simulink model "progetto_smartfarm_luciabrando"  (R2023b)
settings: Solver=VariableStepAuto  StartTime=0.0  StopTime=86400  RelTol=1e-3
libraries: simulink x1
settings Model: Creator=lucia  LastModifiedBy=lucia

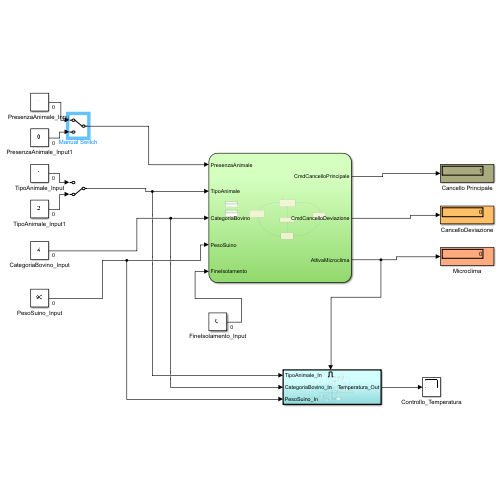
[thumbnail: Simulink's stored preview of the top-level diagram]
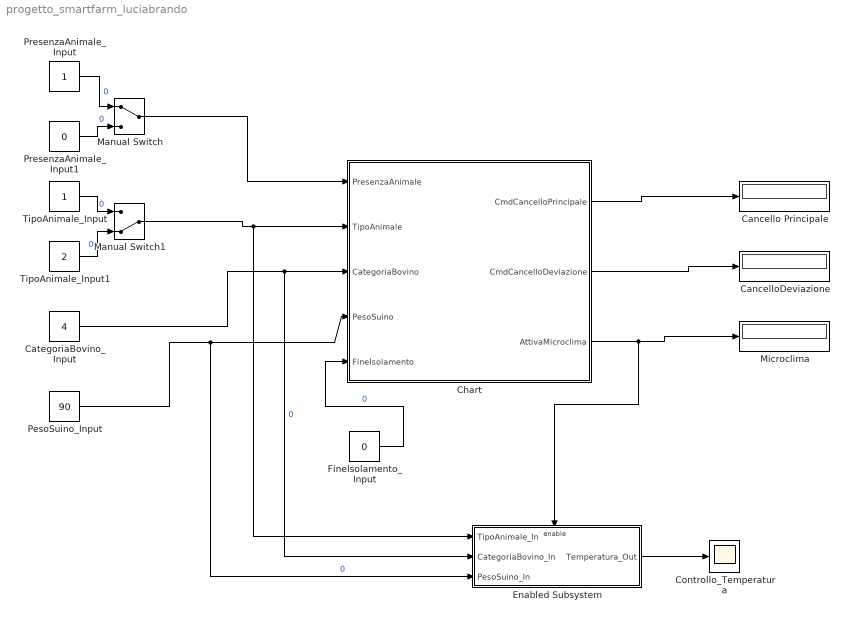
== system progetto_smartfarm_luciabrando ==
  Cancello Principale : Display
  CancelloDeviazione : Display
  CategoriaBovino_Input : Constant  Value=4  OutDataTypeStr=int32
  Chart : Stateflow chart  TreatAsAtomicUnit=on
  Controllo_Temperatura : Scope
  Enabled Subsystem : Subsystem  TreatAsAtomicUnit=on
  FineIsolamento_Input : Constant  Value=0  OutDataTypeStr=boolean
  Manual Switch : ManualSwitch
  Manual Switch1 : ManualSwitch  CurrentSetting=0
  Microclima : Display
  PesoSuino_Input : Constant  Value=90
  PresenzaAnimale_Input : Constant  OutDataTypeStr=boolean
  PresenzaAnimale_Input1 : Constant  Value=0  OutDataTypeStr=boolean
  TipoAnimale_Input : Constant  OutDataTypeStr=int32
  TipoAnimale_Input1 : Constant  Value=2  OutDataTypeStr=int32
  wires:
  Chart/1(CmdCancelloPrincipale) -> Cancello Principale/1
  Chart/2(CmdCancelloDeviazione) -> CancelloDeviazione/1
  PresenzaAnimale_Input/1 -> Manual Switch/1  "0"
  PresenzaAnimale_Input1/1 -> Manual Switch/2  "0"
  Manual Switch/1 -> Chart/1(PresenzaAnimale)
  TipoAnimale_Input/1 -> Manual Switch1/1  "0"
  TipoAnimale_Input1/1 -> Manual Switch1/2  "0"
  Manual Switch1/1 -> Enabled Subsystem/1(TipoAnimale_In), Chart/2(TipoAnimale)
  CategoriaBovino_Input/1 -> Enabled Subsystem/2(CategoriaBovino_In), Chart/3(CategoriaBovino)  "0"
  FineIsolamento_Input/1 -> Chart/5(FineIsolamento)  "0"
  PesoSuino_Input/1 -> Enabled Subsystem/3(PesoSuino_In), Chart/4(PesoSuino)  "0"
  Chart/3(AttivaMicroclima) -> Enabled Subsystem/Enable, Microclima/1
  Enabled Subsystem/1(Temperatura_Out) -> Controllo_Temperatura/1

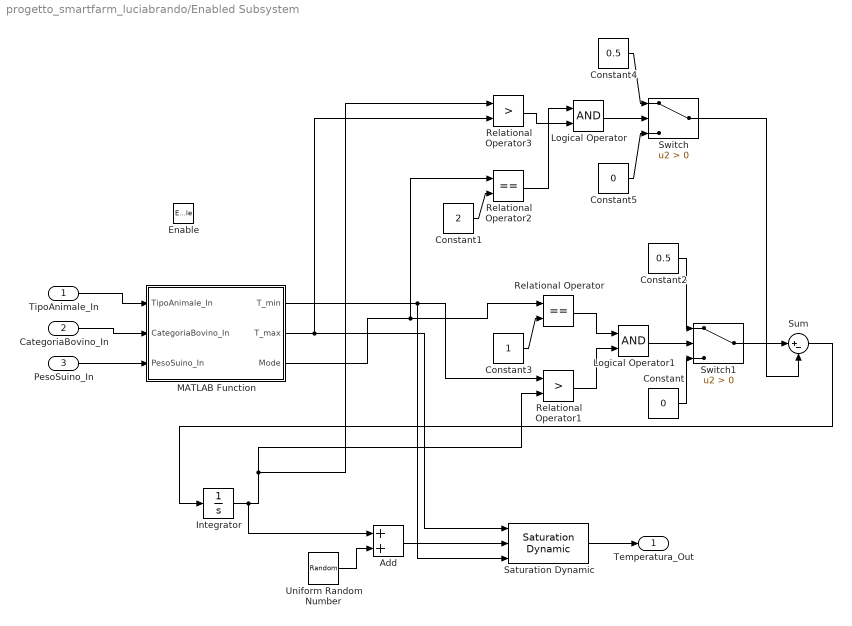
== system progetto_smartfarm_luciabrando/Enabled Subsystem ==
  TipoAnimale_In : Inport
  CategoriaBovino_In : Inport  Port=2
  PesoSuino_In : Inport  Port=3
  Enable : EnablePort
  Add : Sum
  Constant : Constant  Value=0
  Constant1 : Constant  Value=2
  Constant2 : Constant  Value=0.5
  Constant3 : Constant
  Constant4 : Constant  Value=0.5
  Constant5 : Constant  Value=0
  Integrator : Integrator  InitialCondition=20
  Logical Operator : Logic  AllPortsSameDT=off  OutDataTypeStr=boolean
  Logical Operator1 : Logic  AllPortsSameDT=off  OutDataTypeStr=boolean
  MATLAB Function : MATLAB Function  TreatAsAtomicUnit=on
  Relational Operator : RelationalOperator  Operator===  OutDataTypeStr=boolean  RndMeth=Simplest  InputSameDT=off
  Relational Operator1 : RelationalOperator  Operator=>  OutDataTypeStr=boolean  RndMeth=Simplest  InputSameDT=off
  Relational Operator2 : RelationalOperator  Operator===  OutDataTypeStr=boolean  RndMeth=Simplest  InputSameDT=off
  Relational Operator3 : RelationalOperator  Operator=>  OutDataTypeStr=boolean  RndMeth=Simplest  InputSameDT=off
  Saturation Dynamic : simulink/Discontinuities/Saturation Dynamic  OutMin=[]  OutMax=[]  OutDataTypeStr=Inherit: Same as second input  OutDataType=fixdt(1, 16)  OutScaling=2^-10  DoSatur=off
  Sum : Sum  Inputs=|+-
  Switch : Switch  Criteria=u2 > Threshold  SaturateOnIntegerOverflow=off  InputSameDT=off
  Switch1 : Switch  Criteria=u2 > Threshold  SaturateOnIntegerOverflow=off  InputSameDT=off
  Uniform Random Number : UniformRandomNumber  SampleTime=1800
  Temperatura_Out : Outport  InitialOutput=20
  wires:
  TipoAnimale_In/1 -> MATLAB Function/1(TipoAnimale_In)
  CategoriaBovino_In/1 -> MATLAB Function/2(CategoriaBovino_In)
  PesoSuino_In/1 -> MATLAB Function/3(PesoSuino_In)
  Sum/1 -> Integrator/1
  Integrator/1 -> Add/1, Relational Operator1/2, Relational Operator3/1
  MATLAB Function/3(Mode) -> Relational Operator/1, Relational Operator2/1
  Constant3/1 -> Relational Operator/2
  MATLAB Function/1(T_min) -> Saturation Dynamic/3, Relational Operator1/1
  Relational Operator/1 -> Logical Operator1/1
  Relational Operator1/1 -> Logical Operator1/2
  Logical Operator1/1 -> Switch1/2
  Constant2/1 -> Switch1/1
  Constant/1 -> Switch1/3
  Switch1/1 -> Sum/1
  Constant1/1 -> Relational Operator2/2
  MATLAB Function/2(T_max) -> Saturation Dynamic/1, Relational Operator3/2
  Relational Operator2/1 -> Logical Operator/1
  Relational Operator3/1 -> Logical Operator/2
  Logical Operator/1 -> Switch/2
  Constant4/1 -> Switch/1
  Constant5/1 -> Switch/3
  Switch/1 -> Sum/2
  Uniform Random Number/1 -> Add/2
  Add/1 -> Saturation Dynamic/2
  Saturation Dynamic/1 -> Temperatura_Out/1

== matlab function progetto_smartfarm_luciabrando/Enabled Subsystem/MATLAB Function ==
  data: TipoAnimale_In input; CategoriaBovino_In input; PesoSuino_In input; T_min output; T_max output; Mode output
function [T_min, T_max, Mode] = Controllo_Climatico(TipoAnimale_In, CategoriaBovino_In, PesoSuino_In)
    % comandi spenti
    T_min = 30;
    T_max = 30;
    Mode = 0;

    % logica bovini
    if TipoAnimale_In == 1
        if CategoriaBovino_In == 1 || CategoriaBovino_In == 2 || CategoriaBovino_In == 3
            T_min = -6;
            T_max = -4;
            Mode = 2;
        elseif CategoriaBovino_In == 4
            T_min = 29;
            T_max = 32;
            Mode = 1;
        end

    % logica suini
    elseif TipoAnimale_In == 2
        if PesoSuino_In < 50.0
            T_min = 25;
            T_max = 30;
            Mode = 1;
        elseif PesoSuino_In > 85.0
            T_min = 10;
            T_max = 14;
            Mode = 2;
        end
    end
end

== stateflow chart progetto_smartfarm_luciabrando/Chart ==
  state ATTESA
    entry:
    CmdCancelloPrincipale = true;
    CmdCancelloDeviazione = false;
    AttivaMicroclima = false;
  state ISOLAMENTO
    exit:
    CmdCancelloDeviazione = false;
    AttivaMicroclima = false;
  state IDENTIFICAZIONE
  state PASSAGGIO
    entry:
    CmdCancelloPrincipale = true;
  state DECISIONE
  (default) -> ATTESA
  ISOLAMENTO -> ATTESA : [FineIsolamento]
  ATTESA -> IDENTIFICAZIONE : [PresenzaAnimale]/{CmdCancelloPrincipale = false}
  PASSAGGIO -> ATTESA : [after(5,sec)]
  DECISIONE -> ISOLAMENTO [order 2] : [IsBovinoInLista() || IsSuinoInLista()] /{CmdCancelloDeviazione = true; AttivaMicroclima = true }
  IDENTIFICAZIONE -> DECISIONE : [after(10, sec)]
  DECISIONE -> PASSAGGIO [order 1] : [(IsBovinoInLista() || IsSuinoInLista()) == false]/{CmdCancelloPrincipale = true}
  data: inLista function_output; inLista function_output; PresenzaAnimale input boolean; TipoAnimale input int32; CategoriaBovino input int32; PesoSuino input double; FineIsolamento input boolean; CmdCancelloPrincipale output boolean; CmdCancelloDeviazione output boolean; AttivaMicroclima output boolean
  function inLista = IsBovinoInLista:
    | function inLista = IsBovinoInLista()
    |     % Variabili di input
    |     coder.extrinsic('TipoAnimale', 'CategoriaBovino');
    | 
    |     inLista = false; % Default
    | 
    |     if TipoAnimale == 1 % È un bovino
    |         if CategoriaBovino == 1 || ... % Alta Produzione
    |            CategoriaBovino == 2 || ... % Post-Parto
    |            CategoriaBovino == 3 || ... % Gravidanza
    |            CategoriaBovino == 4        % Vitello Giovane
    | 
    |             inLista = true;
    |         end
    |     end
    | end
  function inLista = IsSuinoInLista:
    | function inLista = IsSuinoInLista()
    |     coder.extrinsic('TipoAnimale', 'PesoSuino');
    | 
    |     inLista = false; % Default
    | 
    |     if TipoAnimale == 2 % È un suino
    |         % Condizioni: < 50 kg oppure > 85 kg
    |         if PesoSuino < 50.0 || PesoSuino > 85.0 
    |             inLista = true;
    |         end
    |     end
    | end
